simulink model "IMPLICIT_2ODE_EX5_sim"  (R2019b)
settings: Solver=VariableStepAuto  StartTime=0  StopTime=1  RelTol=1e-3
settings Model: Creator=sulaymon.eshkabilov  LastModifiedBy=sulaymon.eshkabilov

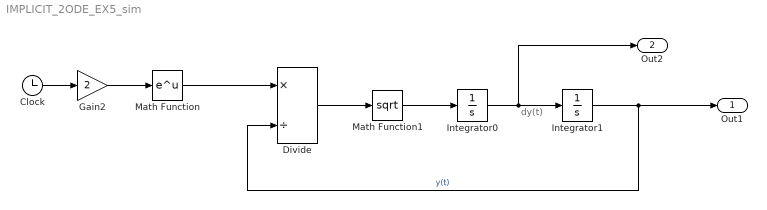
== system IMPLICIT_2ODE_EX5_sim ==
  note: dy(t)
  Clock : Clock
  Divide : Product  Inputs=*/
  Gain2 : Gain  Gain=2
  Integrator0 : Integrator
  Integrator1 : Integrator  InitialCondition=.001
  Math Function : Math  SaturateOnIntegerOverflow=on
  Math Function1 : Math  Operator=sqrt  SaturateOnIntegerOverflow=on
  Out1 : Outport
  Out2 : Outport  Port=2
  wires:
  Integrator0/1 -> Out2/1, Integrator1/1
  Divide/1 -> Math Function1/1
  Gain2/1 -> Math Function/1
  Math Function1/1 -> Integrator0/1
  Integrator1/1 -> Out1/1, Divide/2  "y(t)"
  Math Function/1 -> Divide/1
  Clock/1 -> Gain2/1
